simulink model "second_simu"  (Simulink 7.5)
settings: Solver=ode45  StartTime=0.0  StopTime=10  RelTol=1e-3
libraries: cstblocks x1
settings Model: Creator=N4-MAT-14  LastModifiedBy=N4-MAT-14

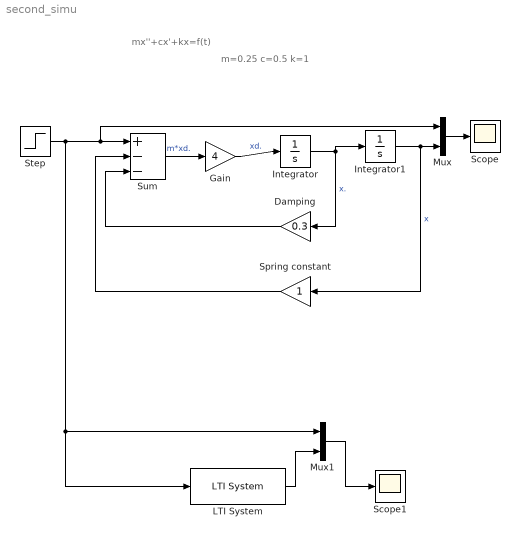
== system second_simu ==
  note: mx''+cx'+kx=f(t)
  note: m=0.25
      | c=0.5
      | k=1
  "Damping " : Gain  Gain=0.3  ParameterDataType=fixdt(1, 16)  ParameterScaling=2^0  OutDataType=fixdt(1, 16)  OutScaling=2^0
  Gain : Gain  Gain=4  ParameterDataType=fixdt(1, 16)  ParameterScaling=2^0  OutDataType=fixdt(1, 16)  OutScaling=2^0
  Integrator : Integrator
  Integrator1 : Integrator
  LTI System : cstblocks/LTI System  SystemSampleTime=-1  sys=tf(2,[2 2])  IC=[]
  Mux : Mux  Inputs=2
  Mux1 : Mux  Inputs=2
  Scope : Scope
      settings: MaxDataPoints=50000
  Scope1 : Scope
  Spring constant : Gain  ParameterDataType=fixdt(1, 16)  ParameterScaling=2^0  OutDataType=fixdt(1, 16)  OutScaling=2^0
  Step : Step  After=3  SampleTime=0
  Sum : Sum  Inputs=+--  OutDataType=fixdt(1, 16)  OutScaling=2^0
  wires:
  Sum/1 -> Gain/1  "m*xd."
  Integrator1/1 -> Spring constant/1, Mux/2  "x"
  Gain/1 -> Integrator/1  "xd."
  Integrator/1 -> Integrator1/1, "Damping "/1  "x."
  "Damping "/1 -> Sum/3
  Spring constant/1 -> Sum/2
  Step/1 -> Sum/1, Mux/1, LTI System/1, Mux1/1
  Mux/1 -> Scope/1
  LTI System/1 -> Mux1/2
  Mux1/1 -> Scope1/1
